simulink model "PD_Control"  (R2021b)
settings: Solver=VariableStepAuto  StartTime=0.0  StopTime=4  RelTol=1e-3
values from neighbouring files (symbols this model uses):
  Gd = -0.1    [Experiment_1.m]
  Gp = -10    [Experiment_1.m]
  s1 = N*Kb    (= 1.27479706572)    [Experiment_1.m]
  s2 = (Jeq/(N*Ktau))*Rm    (= 0.0375418581694)    [Experiment_1.m]
  s3 = (Jeq/(N*Ktau))*Lm    (= 3.71507971468e-06)    [Experiment_1.m]
settings Model: Creator=William Watkins  LastModifiedBy=William Watkins

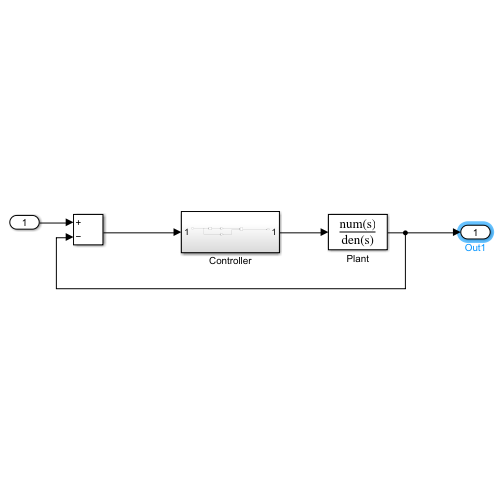
[thumbnail: Simulink's stored preview of the top-level diagram]
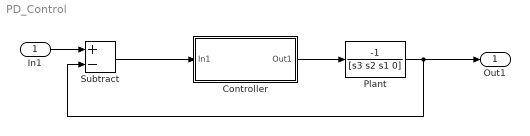
== system PD_Control ==
  In1 : Inport
  Controller : Subsystem
  Plant : TransferFcn  Numerator=[0 0 0 -1]  Denominator=[s3 s2 s1 0]
  Subtract : Sum  Inputs=+-
  Out1 : Outport
  wires:
  Controller/1(Out1) -> Plant/1
  Plant/1 -> Out1/1, Subtract/2
  In1/1 -> Subtract/1
  Subtract/1 -> Controller/1(In1)

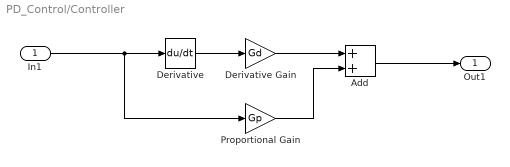
== system PD_Control/Controller ==
  In1 : Inport
  Add : Sum
  Derivative : Derivative
  Derivative Gain : Gain  Gain=Gd
  Proportional Gain : Gain  Gain=Gp
  Out1 : Outport
  wires:
  In1/1 -> Proportional Gain/1, Derivative/1
  Derivative/1 -> Derivative Gain/1
  Derivative Gain/1 -> Add/1
  Proportional Gain/1 -> Add/2
  Add/1 -> Out1/1
